simulink library "sfWorkshop_libs"  (Simulink 7.3)
settings: Solver=ode45  SolverMode=SingleTasking  StartTime=0.0  StopTime=10.0  RelTol=1e-3
undefined symbols (not defined in the file): h0, k, r2h
libraries: fl_lib x12, nesl_utility x6, sfWorkshop_libs x3, aerolibanimutils x1
settings Model: Creator=wcampbel  LastModifiedBy=johnl

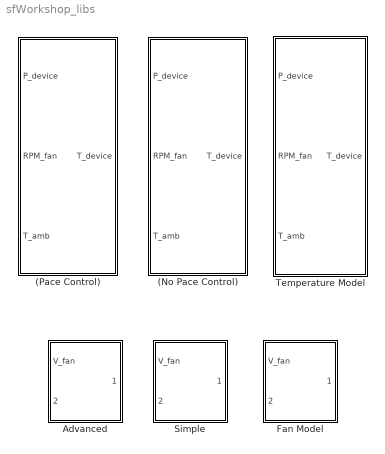
== system sfWorkshop_libs ==
  (No Pace Control) : Subsystem
  (Pace Control) : Subsystem
  Advanced : Subsystem
  Fan Model : Subsystem  BlockChoice=Advanced
      settings: TemplateBlock=self  MemberBlocks=Advanced,Simple
  Simple : Subsystem
  Temperature Model : Subsystem  BlockChoice=(No Pace Control)
      settings: TemplateBlock=self  MemberBlocks=(No Pace Control),(Pace Control)

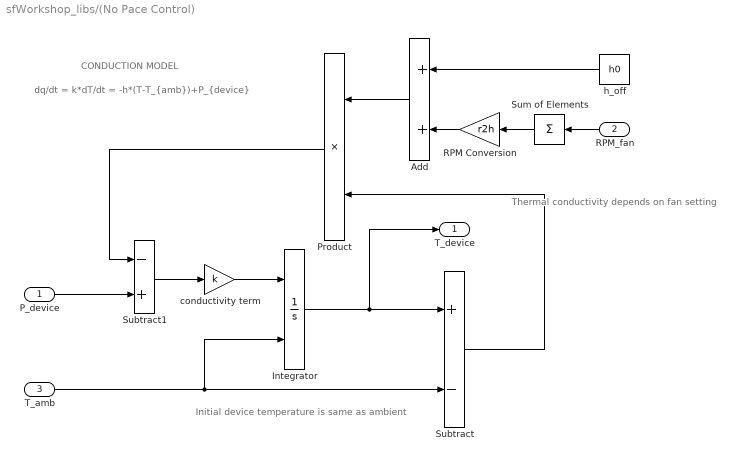
== system sfWorkshop_libs/(No Pace Control) ==
  note: Thermal conductivity
      | depends on fan setting
  note: CONDUCTION MODEL
  note: dq/dt = k*dT/dt = -h*(T-T_{amb})+P_{device}
  note: Initial device temperature
      | is same as ambient
  P_device : Inport  OutDataType=sfix(16)  OutScaling=2^0
  RPM_fan : Inport  Port=2  OutDataType=sfix(16)  OutScaling=2^0
  T_amb : Inport  Port=3  OutDataType=sfix(16)  OutScaling=2^0
  Add : Sum  OutDataType=sfix(16)  OutScaling=2^-10
  Integrator : Integrator  InitialConditionSource=external
  Product : Product  OutDataType=sfix(16)  OutScaling=2^0  RndMeth=Zero
  RPM Conversion : Gain  Gain=r2h  ParameterDataType=sfix(16)  ParameterScaling=2^0  OutDataType=sfix(16)  OutScaling=2^0
  Subtract : Sum  Inputs=+-  OutDataType=sfix(16)  OutScaling=2^-10
  Subtract1 : Sum  Inputs=-+  OutDataType=sfix(16)  OutScaling=2^-10
  Sum of Elements : Sum  Inputs=+  OutDataType=sfix(16)  OutScaling=2^-10
  conductivity term : Gain  Gain=k  ParameterDataType=sfix(16)  ParameterScaling=2^0  OutDataType=sfix(16)  OutScaling=2^0
  h_off : Constant  Value=h0  OutDataType=sfix(16)  OutScaling=2^0
  T_device : Outport  OutDataType=sfix(16)  OutScaling=2^0
  wires:
  Sum of Elements/1 -> RPM Conversion/1
  h_off/1 -> Add/1
  RPM Conversion/1 -> Add/2
  Add/1 -> Product/1
  RPM_fan/1 -> Sum of Elements/1
  Product/1 -> Subtract1/1
  Subtract/1 -> Product/2
  conductivity term/1 -> Integrator/1
  P_device/1 -> Subtract1/2
  T_amb/1 -> Integrator/2, Subtract/2
  Subtract1/1 -> conductivity term/1
  Integrator/1 -> T_device/1, Subtract/1

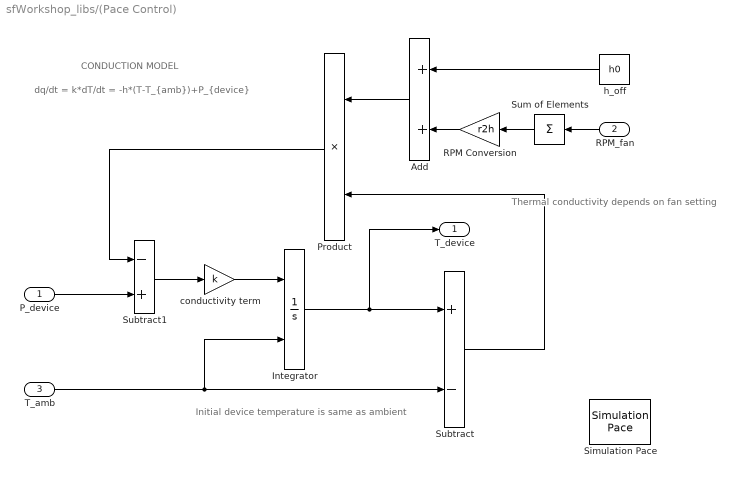
== system sfWorkshop_libs/(Pace Control) ==
  note: Initial device temperature
      | is same as ambient
  note: dq/dt = k*dT/dt = -h*(T-T_{amb})+P_{device}
  note: CONDUCTION MODEL
  note: Thermal conductivity
      | depends on fan setting
  P_device : Inport  OutDataType=sfix(16)  OutScaling=2^0
  RPM_fan : Inport  Port=2  OutDataType=sfix(16)  OutScaling=2^0
  T_amb : Inport  Port=3  OutDataType=sfix(16)  OutScaling=2^0
  Add : Sum  OutDataType=sfix(16)  OutScaling=2^-10
  Integrator : Integrator  InitialConditionSource=external
  Product : Product  OutDataType=sfix(16)  OutScaling=2^0  RndMeth=Zero
  RPM Conversion : Gain  Gain=r2h  ParameterDataType=sfix(16)  ParameterScaling=2^0  OutDataType=sfix(16)  OutScaling=2^0
  Simulation Pace : aerolibanimutils/Simulation Pace  SimulationPace=100  SleepMode=MATLAB Thread  OutputPaceError=off  SampleTime=1/30
      settings: AttributesFormatString=%<SimulationPace> sec/sec
  Subtract : Sum  Inputs=+-  OutDataType=sfix(16)  OutScaling=2^-10
  Subtract1 : Sum  Inputs=-+  OutDataType=sfix(16)  OutScaling=2^-10
  Sum of Elements : Sum  Inputs=+  OutDataType=sfix(16)  OutScaling=2^-10
  conductivity term : Gain  Gain=k  ParameterDataType=sfix(16)  ParameterScaling=2^0  OutDataType=sfix(16)  OutScaling=2^0
  h_off : Constant  Value=h0  OutDataType=sfix(16)  OutScaling=2^0
  T_device : Outport  OutDataType=sfix(16)  OutScaling=2^0
  wires:
  Integrator/1 -> Subtract/1, T_device/1
  Subtract1/1 -> conductivity term/1
  T_amb/1 -> Subtract/2, Integrator/2
  P_device/1 -> Subtract1/2
  conductivity term/1 -> Integrator/1
  Subtract/1 -> Product/2
  Product/1 -> Subtract1/1
  RPM_fan/1 -> Sum of Elements/1
  Add/1 -> Product/1
  RPM Conversion/1 -> Add/2
  h_off/1 -> Add/1
  Sum of Elements/1 -> RPM Conversion/1

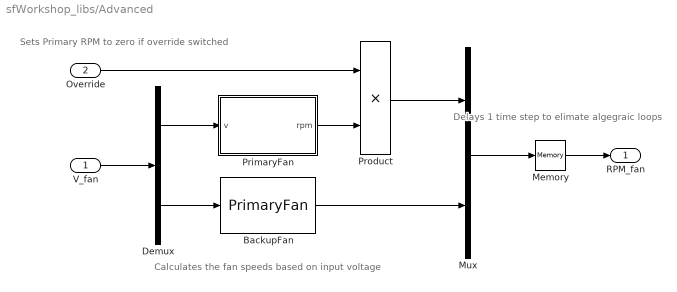
== system sfWorkshop_libs/Advanced ==
  note: Sets Primary RPM to
      | zero if override switched
  note: Calculates the fan speeds
      | based on input voltage
  note: Delays 1 time step to
      | elimate algegraic loops
  V_fan : Inport
  Override : Inport  Port=2
  BackupFan : sfWorkshop_libs/Advanced/PrimaryFan  SystemSampleTime=-1
  Demux : Demux  Outputs=2
  Memory : Memory
  Mux : Mux  Inputs=2
  PrimaryFan : Subsystem
  Product : Product  OutDataType=sfix(16)  OutScaling=2^0  RndMeth=Zero
  RPM_fan : Outport
  wires:
  Mux/1 -> Memory/1
  V_fan/1 -> Demux/1
  Demux/2 -> BackupFan/1
  Demux/1 -> PrimaryFan/1(v)
  BackupFan/1 -> Mux/2
  Product/1 -> Mux/1
  PrimaryFan/1(rpm) -> Product/2
  Override/1 -> Product/1
  Memory/1 -> RPM_fan/1

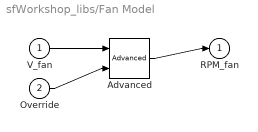
== system sfWorkshop_libs/Fan Model ==
  V_fan : Inport
  Override : Inport  Port=2
  Advanced : sfWorkshop_libs/Advanced  SystemSampleTime=-1
  RPM_fan : Outport
  wires:
  V_fan/1 -> Advanced/1
  Override/1 -> Advanced/2
  Advanced/1 -> RPM_fan/1

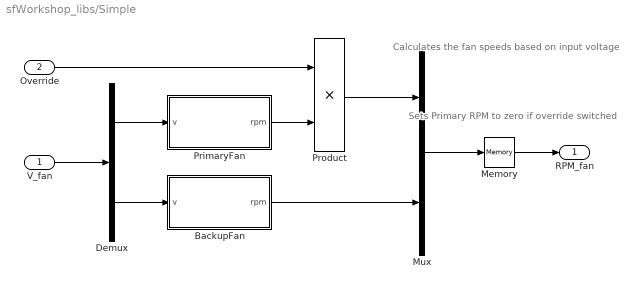
== system sfWorkshop_libs/Simple ==
  note: Calculates the fan speeds
      | based on input voltage
  note: Sets Primary RPM to
      | zero if override switched
  V_fan : Inport
  Override : Inport  Port=2
  BackupFan : Subsystem
  Demux : Demux  Outputs=2
  Memory : Memory
  Mux : Mux  Inputs=2
  PrimaryFan : Subsystem
  Product : Product  OutDataType=sfix(16)  OutScaling=2^0  RndMeth=Zero
  RPM_fan : Outport
  wires:
  Override/1 -> Product/1
  PrimaryFan/1(rpm) -> Product/2
  Product/1 -> Mux/1
  BackupFan/1(rpm) -> Mux/2
  Demux/1 -> PrimaryFan/1(v)
  Demux/2 -> BackupFan/1(v)
  V_fan/1 -> Demux/1
  Mux/1 -> Memory/1
  Memory/1 -> RPM_fan/1

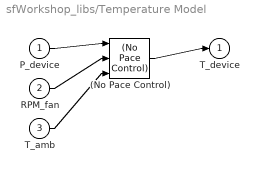
== system sfWorkshop_libs/Temperature Model ==
  P_device : Inport
  RPM_fan : Inport  Port=2
  T_amb : Inport  Port=3
  (No Pace Control) : sfWorkshop_libs/(No Pace Control)  SystemSampleTime=-1
  T_device : Outport
  wires:
  P_device/1 -> (No Pace Control)/1
  RPM_fan/1 -> (No Pace Control)/2
  T_amb/1 -> (No Pace Control)/3
  (No Pace Control)/1 -> T_device/1

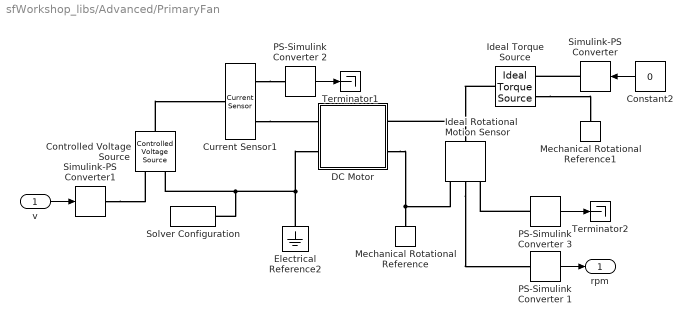
== system sfWorkshop_libs/Advanced/PrimaryFan ==
  v : Inport
  Constant2 : Constant  Value=0  OutDataType=sfix(16)  OutScaling=2^0
  Controlled Voltage Source : fl_lib/Electrical/Electrical Sources/Controlled Voltage Source  DialogController=NetworkEngine.DynNeDlgSource  SystemSampleTime=-1  i_Log=off  v_Log=off  LocalVarNames=|i|v  LocalVarDescs=|i|v  LocalVarLogging=[0 0]
  Current Sensor1 : fl_lib/Electrical/Electrical Sensors/Current Sensor  DialogController=NetworkEngine.DynNeDlgSource  SystemSampleTime=-1  i1_Log=off  v1_Log=off  LocalVarNames=|i1|v1  LocalVarDescs=|i1|v1  LocalVarLogging=[0 0]
  DC Motor : Subsystem
  Electrical Reference2 : fl_lib/Electrical/Electrical Elements/Electrical Reference  DialogController=NetworkEngine.DynNeDlgSource  SystemSampleTime=-1  i_Log=off  LocalVarNames=|i  LocalVarDescs=|i  LocalVarLogging=[]
  Ideal Rotational Motion Sensor : fl_lib/Mechanical/Mechanical Sensors/Ideal Rotational Motion Sensor  DialogController=NetworkEngine.DynNeDlgSource  SystemSampleTime=-1  offset=0 rad  w_Log=off  t_Log=off  phi_Log=off  LocalVarNames=|w|t|phi  LocalVarDescs=|w|t|phi  LocalVarLogging=[]
  Ideal Torque Source : fl_lib/Mechanical/Mechanical Sources/Ideal Torque Source  DialogController=NetworkEngine.DynNeDlgSource  SystemSampleTime=-1  w_Log=off  t_Log=off  LocalVarNames=|w|t  LocalVarDescs=|w|t  LocalVarLogging=[0 0]
  Mechanical Rotational Reference : fl_lib/Mechanical/Rotational Elements/Mechanical Rotational Reference  DialogController=NetworkEngine.DynNeDlgSource  SystemSampleTime=-1  t_Log=off  LocalVarNames=|t  LocalVarDescs=|t  LocalVarLogging=[]
  Mechanical Rotational Reference1 : fl_lib/Mechanical/Rotational Elements/Mechanical Rotational Reference  DialogController=NetworkEngine.DynNeDlgSource  SystemSampleTime=-1  t_Log=off  LocalVarNames=|t  LocalVarDescs=|t  LocalVarLogging=[]
  PS-Simulink Converter 1 : nesl_utility/PS-Simulink Converter  DialogController=NetworkEngine.DynNeUtilDlgSource  SystemSampleTime=-1  PhysicalDomain=network_engine_domain  LeftPortType=input  RightPortType=output  SubClassName=ps_output  Unit=rpm  AffineConversion=off
  PS-Simulink Converter 2 : nesl_utility/PS-Simulink Converter  DialogController=NetworkEngine.DynNeUtilDlgSource  SystemSampleTime=-1  PhysicalDomain=network_engine_domain  LeftPortType=input  RightPortType=output  SubClassName=ps_output  Unit=1  AffineConversion=off
  PS-Simulink Converter 3 : nesl_utility/PS-Simulink Converter  DialogController=NetworkEngine.DynNeUtilDlgSource  SystemSampleTime=-1  PhysicalDomain=network_engine_domain  LeftPortType=input  RightPortType=output  SubClassName=ps_output  Unit=deg  AffineConversion=off
  Simulink-PS Converter : nesl_utility/Simulink-PS Converter  DialogController=NetworkEngine.DynNeUtilDlgSource  SystemSampleTime=-1  PhysicalDomain=network_engine_domain  LeftPortType=input  RightPortType=output  SubClassName=ps_input  Unit=1  AffineConversion=off  InputFilterTimeConstant=.001  UdotUserProvided=0
  Simulink-PS Converter1 : nesl_utility/Simulink-PS Converter  DialogController=NetworkEngine.DynNeUtilDlgSource  SystemSampleTime=-1  PhysicalDomain=network_engine_domain  LeftPortType=input  RightPortType=output  SubClassName=ps_input  Unit=1  AffineConversion=off  InputFilterTimeConstant=.001  UdotUserProvided=0
  Solver Configuration : nesl_utility/Solver Configuration  DialogController=NetworkEngine.DynNeUtilDlgSource  SystemSampleTime=-1  PhysicalDomain=network_engine_domain  LeftPortType=input  RightPortType=generic  SubClassName=solver  Accelerate=off  Profile=off  ResidualTolerance=1e-9  MaxNonlinIter=12  MaxModeIter=2  DoFixedCost=off  DoDC=off  LinearAlgebra=Sparse
  Terminator1 : Terminator
  Terminator2 : Terminator
  rpm : Outport
  wires:
  PS-Simulink Converter 3/1 -> Terminator2/1
  PS-Simulink Converter 1/1 -> rpm/1
  v/1 -> Simulink-PS Converter1/1
  Constant2/1 -> Simulink-PS Converter/1
  PS-Simulink Converter 2/1 -> Terminator1/1
  connections:
  PS-Simulink Converter 3/LConn1 -- Ideal Rotational Motion Sensor/RConn3
  Ideal Torque Source/RConn2 -- Mechanical Rotational Reference1/LConn1
  Simulink-PS Converter/RConn1 -- Ideal Torque Source/RConn1
  Ideal Rotational Motion Sensor/RConn2 -- PS-Simulink Converter 1/LConn1
  Ideal Rotational Motion Sensor/RConn1 -- Mechanical Rotational Reference/LConn1 -- DC Motor/RConn2
  Ideal Torque Source/LConn1 -- Ideal Rotational Motion Sensor/LConn1 -- DC Motor/RConn1
  Current Sensor1/RConn2 -- DC Motor/LConn1
  Current Sensor1/RConn1 -- PS-Simulink Converter 2/LConn1
  Controlled Voltage Source/RConn2 -- Electrical Reference2/LConn1 -- DC Motor/LConn2 -- Solver Configuration/RConn1
  Simulink-PS Converter1/RConn1 -- Controlled Voltage Source/RConn1
  Controlled Voltage Source/LConn1 -- Current Sensor1/LConn1

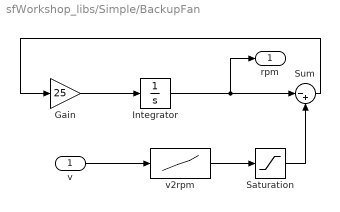
== system sfWorkshop_libs/Simple/BackupFan ==
  v : Inport
  Gain : Gain  Gain=25  ParameterDataType=sfix(16)  ParameterScaling=2^0  OutDataType=sfix(16)  OutScaling=2^0
  Integrator : Integrator
  Saturation : Saturate  UpperLimit=6000  LowerLimit=0  OutDataType=sfix(16)  OutScaling=2^0
  Sum : Sum  Inputs=|-+  OutDataType=sfix(16)  OutScaling=2^0
  v2rpm : Lookup  InputValues=[.75 1]  Table=[2538 6000]  OutDataType=sfix(16)  OutScaling=2^0
  rpm : Outport
  wires:
  Gain/1 -> Integrator/1
  Integrator/1 -> Sum/1, rpm/1
  v/1 -> v2rpm/1
  Sum/1 -> Gain/1
  v2rpm/1 -> Saturation/1
  Saturation/1 -> Sum/2

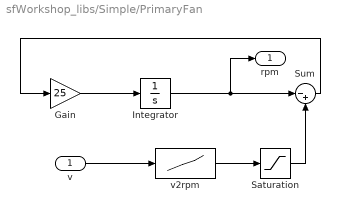
== system sfWorkshop_libs/Simple/PrimaryFan ==
  v : Inport
  Gain : Gain  Gain=25  ParameterDataType=sfix(16)  ParameterScaling=2^0  OutDataType=sfix(16)  OutScaling=2^0
  Integrator : Integrator
  Saturation : Saturate  UpperLimit=6000  LowerLimit=0  OutDataType=sfix(16)  OutScaling=2^0
  Sum : Sum  Inputs=|-+  OutDataType=sfix(16)  OutScaling=2^0
  v2rpm : Lookup  InputValues=[.75 1]  Table=[2538 6000]  OutDataType=sfix(16)  OutScaling=2^0
  rpm : Outport
  wires:
  v2rpm/1 -> Saturation/1
  Sum/1 -> Gain/1
  v/1 -> v2rpm/1
  Integrator/1 -> rpm/1, Sum/1
  Gain/1 -> Integrator/1
  Saturation/1 -> Sum/2

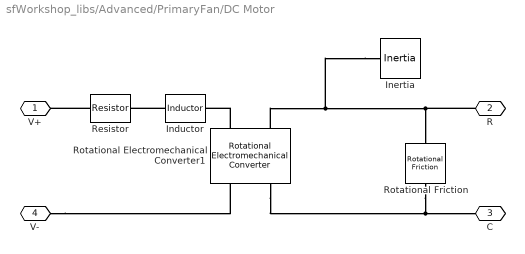
== system sfWorkshop_libs/Advanced/PrimaryFan/DC Motor ==
  Inductor : fl_lib/Electrical/Electrical Elements/Inductor  DialogController=NetworkEngine.DynNeDlgSource  SystemSampleTime=-1  l=12e-6 H  i0=0 A  r=0 Ohm  g=1e-09 1/Ohm  i_Log=off  v_Log=off  i_L_Log=off  LocalVarNames=|i|v|i_L  LocalVarDescs=|i|v|Internal variable for current through inductor term  LocalVarLogging=[0 0 0]
  Inertia : fl_lib/Mechanical/Rotational Elements/Inertia  DialogController=NetworkEngine.DynNeDlgSource  SystemSampleTime=-1  inertia=0.01 g*cm^2  initial_velocity=0 rad/s  t_Log=off  LocalVarNames=|t  LocalVarDescs=|t  LocalVarLogging=0
  Resistor : fl_lib/Electrical/Electrical Elements/Resistor  DialogController=NetworkEngine.DynNeDlgSource  SystemSampleTime=-1  R=3.9*5 Ohm  i_Log=off  v_Log=off  LocalVarNames=|i|v  LocalVarDescs=|i|v  LocalVarLogging=[0 0]
  Rotational Electromechanical Converter1 : fl_lib/Electrical/Electrical Elements/Rotational Electromechanical Converter  DialogController=NetworkEngine.DynNeDlgSource  SystemSampleTime=-1  K=0.072e-3*60/(2*pi) V/(rad/s)  i_Log=off  v_Log=off  t_Log=off  w_Log=off  LocalVarNames=|i|v|t|w  LocalVarDescs=|i|v|t|w  LocalVarLogging=[0 0 0 0]
  Rotational Friction : fl_lib/Mechanical/Rotational Elements/Rotational Friction  DialogController=NetworkEngine.DynNeDlgSource  SystemSampleTime=-1  brkwy_trq=0.02e-3 N*m  Col_trq=0.02e-3 N*m  visc_coef=0 N*m/(rad/s)  trans_coef=10 s/rad  vel_thr=0.1 rad/s  t_Log=off  w_Log=off  LocalVarNames=|t|w  LocalVarDescs=|t|w  LocalVarLogging=[0 0]
  V+ : PMIOPort  Port=1  Side=Left
  R : PMIOPort  Port=2  Side=Right
  C : PMIOPort  Port=3  Side=Right
  V- : PMIOPort  Port=4  Side=Left
  connections:
  Rotational Friction/RConn1 -- C/RConn1 -- Rotational Electromechanical Converter1/RConn2
  Inertia/LConn1 -- R/RConn1 -- Rotational Friction/LConn1 -- Rotational Electromechanical Converter1/LConn2
  Inductor/LConn1 -- Resistor/RConn1
  Resistor/LConn1 -- V+/RConn1
  V-/RConn1 -- Rotational Electromechanical Converter1/RConn1
  Rotational Electromechanical Converter1/LConn1 -- Inductor/RConn1
